simulink model "Sim68BusSg"  (R2020b)
settings: Solver=FixedStepAuto  StartTime=0  StopTime=5  FixedStep=Ts  RelTol=1e-3
values from neighbouring files (symbols this model uses):
  Sbase = 1    [Para.m]    (also in Para_VFM_FFL_Inverter.m; Para_VFM_FFL_Inverter_v2.m)
  Ts = 1/Fs    (= 0.0001)    [Para.m]    (also in Para_VFM_FFL_Inverter.m; Para_VFM_FFL_Inverter_v2.m = 5e-05)
  Vbase = 1    [Para.m]    (also in Para_VFM_FFL_Inverter.m; Para_VFM_FFL_Inverter_v2.m)
  Wbase = 2*pi*50    (= 314.159265359)    [Para.m]    (also in Para_VFM_FFL_Inverter.m; Para_VFM_FFL_Inverter_v2.m)
  Ybase = 1/Zbase    (= 1)    [Para.m]    (also in Para_VFM_FFL_Inverter.m; Para_VFM_FFL_Inverter_v2.m)
  Zbase = Vbase/Ibase    (= 1)    [Para.m]    (also in Para_VFM_FFL_Inverter.m; Para_VFM_FFL_Inverter_v2.m)
undefined symbols (not defined in the file or in its folder): ApparatusDiscreDamping, ApparatusPara, ApparatusPowerFlow, ApparatusType, Fbase, OtherInputs, x_e
libraries: powerlib x223, SimplusGT x86
(part 2 of 2)

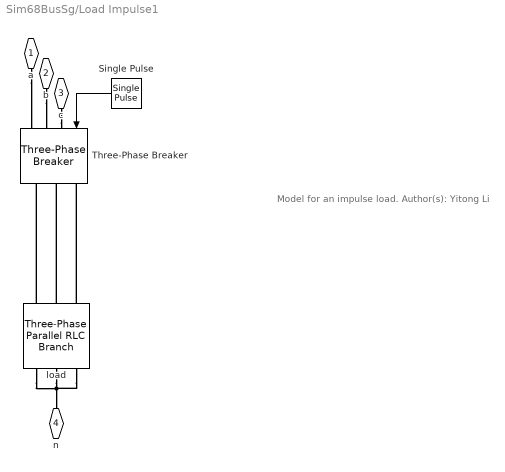
== system Sim68BusSg/Load Impulse1 ==
  note: Model for an impulse load.
      |
      | Author(s): Yitong Li
  Single Pulse : SimplusGT/Single Pulse  t0=t0  dt=dt  Am=1
  Three-Phase Breaker : powerlib/Elements/Three-Phase Breaker  InitialState=open  SwitchA=on  SwitchB=on  SwitchC=on  SwitchTimes="[1/60  5/60]"  External=on  BreakerResistance=1e-9  SnubberResistance=1e6  SnubberCapacitance=inf  Measurements=None
  load : powerlib/Elements/Three-Phase Parallel RLC Branch  LConnTagsString=A|B|C  RConnTagsString=A|B|C  BranchType=R  Resistance=R  Inductance=1  Capacitance=1  Measurements=None
      settings: SourceProductBaseCode=PS
  a : PMIOPort  Side=Left
  b : PMIOPort  Port=2  Side=Left
  c : PMIOPort  Port=3  Side=Left
  n : PMIOPort  Port=4  Side=Right
  wires:
  Single Pulse/1 -> Three-Phase Breaker/1
  connections:
  load/RConn2 -- load/RConn3 -- load/RConn1 -- n/RConn1
  c/RConn1 -- Three-Phase Breaker/LConn1
  b/RConn1 -- Three-Phase Breaker/LConn2
  a/RConn1 -- Three-Phase Breaker/LConn3
  load/LConn1 -- Three-Phase Breaker/RConn3
  load/LConn2 -- Three-Phase Breaker/RConn2
  load/LConn3 -- Three-Phase Breaker/RConn1
